simulink model "Cart_Pendulum_Linearised_a_n9558292"  (R2018a)
settings: Solver=VariableStepAuto  StartTime=0.0  StopTime=10.0  RelTol=1e-3
values from neighbouring files (symbols this model uses):
  g = 9.81    [MainFile_Linearised_a_n9558292.m]    (also in MainFile_Linearised_b_n9558292.m; MainFile_n9558292.m)
  l = 0.2    [MainFile_Linearised_a_n9558292.m]    (also in MainFile_Linearised_b_n9558292.m; MainFile_n9558292.m)
  m = 0.15    [MainFile_Linearised_a_n9558292.m]    (also in MainFile_Linearised_b_n9558292.m; MainFile_n9558292.m)
  Mc = 0.4    [MainFile_Linearised_a_n9558292.m]    (also in MainFile_Linearised_b_n9558292.m; MainFile_n9558292.m)
  stepfa_tilde = 10    [MainFile_Linearised_a_n9558292.m]
  stepia_tilde = 0    [MainFile_Linearised_a_n9558292.m]
  stepta_tilde = 1    [MainFile_Linearised_a_n9558292.m]
  x10a_tilde = 0    [MainFile_Linearised_a_n9558292.m]
  x20a_tilde = pi    (= 3.14159265359)    [MainFile_Linearised_a_n9558292.m]
  x30a_tilde = 0    [MainFile_Linearised_a_n9558292.m]
  x40a_tilde = 0    [MainFile_Linearised_a_n9558292.m]
settings Model: Creator=haidarobeid  LastModifiedBy=haidarobeid
settings DataIOCC: SaveFormat=Array  TimeSaveName=touta_tilde

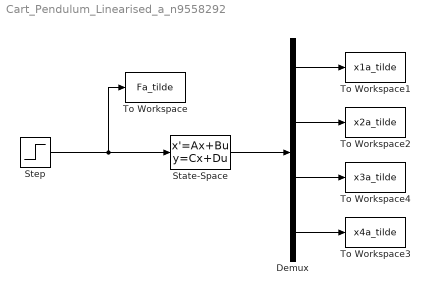
== system Cart_Pendulum_Linearised_a_n9558292 ==
  Demux : Demux
  State-Space : StateSpace  A=[0,0,1,0;0,0,0,1;0,-m*g/Mc,0,0;0,g*(Mc+m)/(l*Mc),0,0]  B=[0;0;1/Mc;-1/(l*Mc)]  C=eye(4)  D=[0; 0; 0 ;0]  InitialCondition=[x10a_tilde;x20a_tilde;x30a_tilde;x40a_tilde]
  Step : Step  Time=stepta_tilde  Before=stepia_tilde  After=stepfa_tilde  SampleTime=0
  To Workspace : ToWorkspace  VariableName=Fa_tilde  SampleTime=-1
  To Workspace1 : ToWorkspace  VariableName=x1a_tilde  SampleTime=-1
  To Workspace2 : ToWorkspace  VariableName=x2a_tilde  SampleTime=-1
  To Workspace3 : ToWorkspace  VariableName=x4a_tilde  SampleTime=-1
  To Workspace4 : ToWorkspace  VariableName=x3a_tilde  SampleTime=-1
  wires:
  State-Space/1 -> Demux/1
  Demux/1 -> To Workspace1/1
  Demux/2 -> To Workspace2/1
  Demux/3 -> To Workspace4/1
  Demux/4 -> To Workspace3/1
  Step/1 -> To Workspace/1, State-Space/1
